simulink model "AerosondA_UAV_6DOF"  (R2021a)
settings: Solver=VariableStepAuto  StartTime=0.0  StopTime=20.0  RelTol=1e-3
InitFcn:
  | %%%%%%%%%%%%%%%%%%%%%%% Airframe Parameters %%%%%%%%%%%%%%%%%%%%%%%%%%%%%%%
  | 
  | m=13.5; % mass(kg)
  | Ix=0.8244; % Inertia along x axis (kg*m^2)
  | Iy=1.135; % Inertia along y axis (kg*m^2)
  | Iz=1.759; % Inertia along z axis (kg*m^2)
  | Ixy=0; % Inertia on xy plane (kg*m^2)
  | Iyz=0; % Inertia on yz plane (kg*m^2)
  | Ixz=0.1204; % Inertia on xz plane (kg*m^2)
  | I=[Ix -Ixy -Ixz;-Ixy Iy -Iyz;-Ixz -Iyz Iz]; % Inertia Matrix
  | S=0.55; % Surface Area (m^2)
  | b=2.8956; % Wingspan (m)
  | c=0.18994; % Chord (m)
  | Sprop=0.2027; % Propeller Surface Area (m^2)
  | k_motor=80; % Motor Constant
  | kTp=0; % Experimental Constant
  | k_omega=0; % Propeller Rotation Constant
  | rho_SL=1.225; % Sea Level air Density(kg/m^3)
  | TrimCondition(1)=-3.0373; % Elevator Trim At 100 m (degree)
  | TrimCondition(2)=0; % Aileron Trim At 100 m (degree)
  | TrimCondition(3)=0; % Rudder Trim At 100 m (degree)
  | TrimCondition(4)=0.45225; % Throttle Trim At 100 m
  | 
  | 
  | 
  | %%%%%%%%%%%%%%%%%%%%% Longitudinal Coefficients %%%%%%%%%%%%%%%%%%%%%%%%%%%
  | 
  | CL0=0.28;
  | CD0=0.03;
  | Cm0=-0.02338;
  | dCLdalpha=3.45;
  | dCDdalpha=0.3;
  | dCmdalpha=-0.38;
  | dCLdq=0;
  | dCDdq=0;
  | dCmdq=-3.6;
  | dCLdsigmaE=-0.36;
  | dCDdsigmaE=0;
  | dCmdsigmaE=-0.5;
  | Cprop=1;
  | M=50;
  | alpha_0=0.4712;
  | epsilon=0.1592;
  | dCDdp=0.0437;
  | dCndsigmaR=-0.032;
  | 
  | 
  | %%%%%%%%%%%%%%%%%%%%%%%% Lateral Coefficients %%%%%%%%%%%%%%%%%%%%%%%%%%%%%
  | 
  | Cy0=0;
  | Cl0=0;
  | Cn0=0;
  | dCydbeta=-0.98;
  | dCldbeta=-0.12;
  | dCndbeta=0.25;
  | dCydp=0;
  | dCldp=-0.26;
  | dCndp=0.022;
  | dCydr=0;
  | dCldr=0.14;
  | dCndr=-0.35;
  | dCydsigmaA=0;
  | dCldsigmaA=0.08;
  | dCndsigmaA=0.06;
  | dCydsigmaR=-0.17;
  | dCldsigmaR=-0.105;
undefined symbols (not defined in the file): TrimCondition
libraries: simulink_extras x3, aerolibutil x1
settings Model: Creator=hasre  LastModifiedBy=hasre

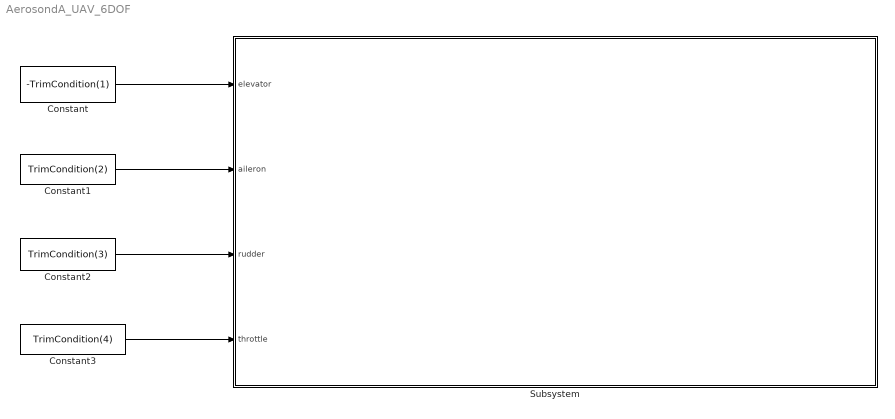
== system AerosondA_UAV_6DOF ==
  Constant : Constant  Value=-TrimCondition(1)
  Constant1 : Constant  Value=TrimCondition(2)
  Constant2 : Constant  Value=TrimCondition(3)
  Constant3 : Constant  Value=TrimCondition(4)
  Subsystem : Subsystem
  wires:
  Constant/1 -> Subsystem/1("elevator ")
  Constant1/1 -> Subsystem/2("aileron ")
  Constant2/1 -> Subsystem/3("rudder ")
  Constant3/1 -> Subsystem/4("throttle ")

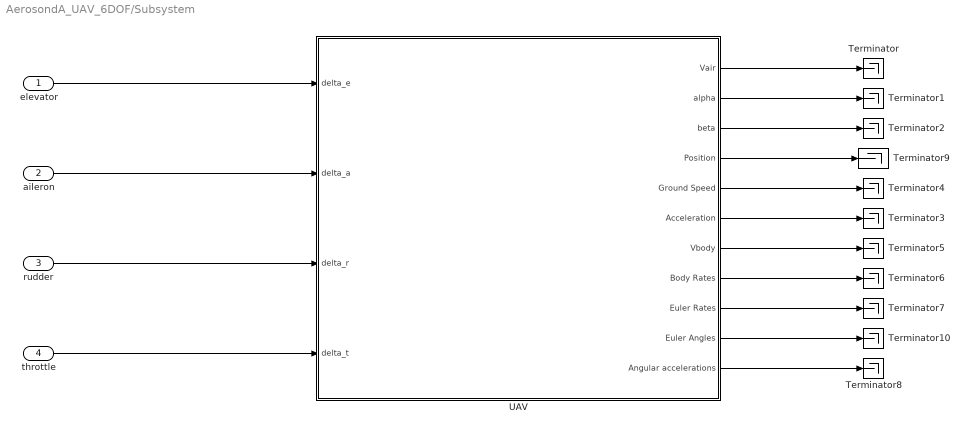
== system AerosondA_UAV_6DOF/Subsystem ==
  "elevator " : Inport
  "aileron " : Inport  Port=2
  "rudder " : Inport  Port=3
  "throttle " : Inport  Port=4
  Terminator{,1..10} (11 alike) : Terminator
  UAV : Subsystem
  wires:
  UAV/8(Body Rates) -> Terminator6/1
  UAV/6(Acceleration) -> Terminator3/1
  UAV/7(Vbody) -> Terminator5/1
  "elevator "/1 -> UAV/1(delta_e)
  UAV/3(beta) -> Terminator2/1
  "aileron "/1 -> UAV/2("delta_a ")
  UAV/4(Position) -> Terminator9/1
  UAV/1(Vair) -> Terminator/1
  UAV/11(Angular accelerations) -> Terminator8/1
  "throttle "/1 -> UAV/4(delta_t)
  UAV/2(alpha) -> Terminator1/1
  UAV/9(Euler Rates) -> Terminator7/1
  "rudder "/1 -> UAV/3(delta_r)
  UAV/5(Ground Speed) -> Terminator4/1
  UAV/10(Euler Angles) -> Terminator10/1

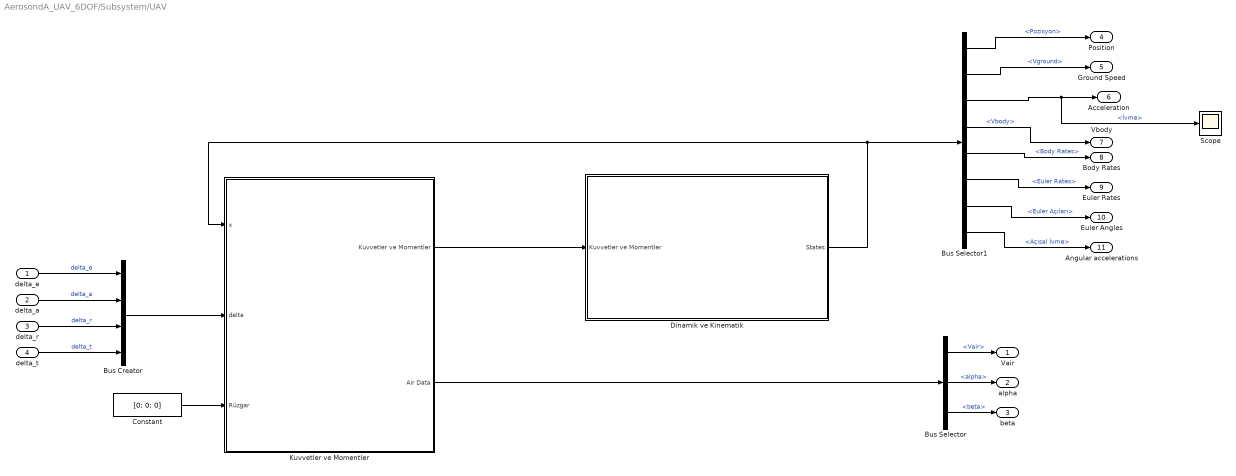
== system AerosondA_UAV_6DOF/Subsystem/UAV ==
  delta_e : Inport
  "delta_a " : Inport  Port=2
  delta_r : Inport  Port=3
  delta_t : Inport  Port=4
  Bus Creator : BusCreator  Inputs=4
  Bus Selector : BusSelector  OutputSignals=Vair,alpha,beta
  Bus Selector1 : BusSelector  OutputSignals=Pozisyon,Vground,İvme,Vbody,Body Rates,Euler Rates,Euler Açıları,Açısal İvme
  Constant : Constant  Value=[0; 0; 0]  VectorParams1D=off
  Dinamik ve Kinematik : Subsystem
  Kuvvetler ve Momentler : Subsystem
  Scope : Scope
  Vair : Outport
  alpha : Outport  Port=2
  beta : Outport  Port=3
  Position : Outport  Port=4
  Ground Speed : Outport  Port=5
  Acceleration : Outport  Port=6
  Vbody : Outport  Port=7
  Body Rates : Outport  Port=8
  Euler Rates : Outport  Port=9
  Euler Angles : Outport  Port=10
  Angular accelerations : Outport  Port=11
  wires:
  Kuvvetler ve Momentler/1(Kuvvetler ve Momentler) -> Dinamik ve Kinematik/1(Kuvvetler ve Momentler)
  delta_r/1 -> Bus Creator/3  "delta_r"
  delta_e/1 -> Bus Creator/1  "delta_e"
  Dinamik ve Kinematik/1(States) -> Kuvvetler ve Momentler/1("x "), Bus Selector1/1
  "delta_a "/1 -> Bus Creator/2  "delta_a"
  delta_t/1 -> Bus Creator/4  "delta_t"
  Bus Selector/2 -> alpha/1  "<alpha>"
  Bus Selector/1 -> Vair/1  "<Vair>"
  Kuvvetler ve Momentler/2(Air Data) -> Bus Selector/1
  Bus Selector/3 -> beta/1  "<beta>"
  Bus Creator/1 -> Kuvvetler ve Momentler/2("delta ")
  Constant/1 -> Kuvvetler ve Momentler/3(Rüzgar)
  Bus Selector1/1 -> Position/1  "<Pozisyon>"
  Bus Selector1/2 -> Ground Speed/1  "<Vground>"
  Bus Selector1/3 -> Scope/1, Acceleration/1  "<İvme>"
  Bus Selector1/4 -> Vbody/1  "<Vbody>"
  Bus Selector1/5 -> Body Rates/1  "<Body Rates>"
  Bus Selector1/6 -> Euler Rates/1  "<Euler Rates>"
  Bus Selector1/7 -> Euler Angles/1  "<Euler Açıları>"
  Bus Selector1/8 -> Angular accelerations/1  "<Açısal İvme>"

== system AerosondA_UAV_6DOF/Subsystem/UAV/Dinamik ve Kinematik ==
  Kuvvetler ve Momentler : Inport
  6 DOF Model : Subsystem
  Bus Creator : BusCreator  Inputs=9
  Bus Selector : BusSelector  OutputSignals=Kuvvetler,Momentler
  States : Outport
  wires:
  6 DOF Model/7(İvme (m/s2)) -> Bus Creator/7  "İvme"
  6 DOF Model/4(ωb (rad/s)) -> Bus Creator/4  "Body Rates"
  6 DOF Model/8(Earth Fixed Pos. (m)) -> Bus Creator/8  "Pozisyon"
  6 DOF Model/9(DCMvb) -> Bus Creator/9  "Euler Matrix"
  6 DOF Model/1("ϕ θ ψ (rad)  ") -> Bus Creator/1  "Euler Açıları"
  6 DOF Model/3("Vb (m/s) ") -> Bus Creator/3  "Vbody"
  6 DOF Model/5(dωb/dt) -> Bus Creator/5  "Açısal İvme"
  6 DOF Model/6(Vg) -> Bus Creator/6  "Vground"
  Kuvvetler ve Momentler/1 -> Bus Selector/1
  Bus Selector/2 -> 6 DOF Model/2(Moment)  "<Momentler>"
  Bus Selector/1 -> 6 DOF Model/1(Kuvvet)  "<Kuvvetler>"
  6 DOF Model/2(ϕ θ ψ rates (rad/s)) -> Bus Creator/2  "Euler Rates"
  Bus Creator/1 -> States/1

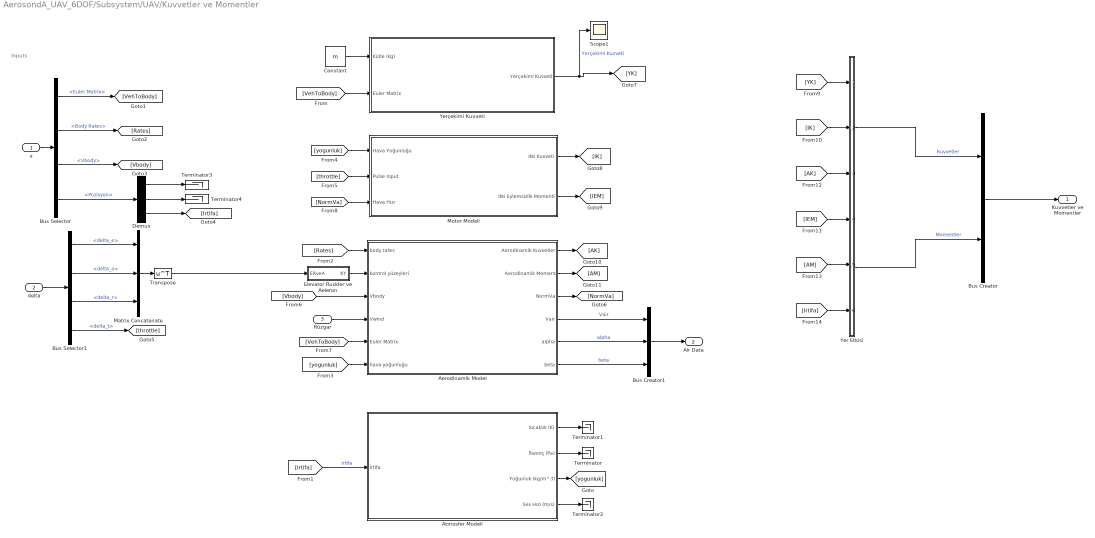
== system AerosondA_UAV_6DOF/Subsystem/UAV/Kuvvetler ve Momentler ==
  note: Inputs
  "x " : Inport
  "delta " : Inport  Port=2
  Rüzgar : Inport  Port=3
  Aerodinamik Model : Subsystem
  Atmosfer Modeli : Subsystem
  Bus Creator : BusCreator  Inputs=2
  Bus Creator1 : BusCreator  Inputs=3
  Bus Selector : BusSelector  OutputSignals=Euler Matrix,Body Rates,Vbody,Pozisyon
  Bus Selector1 : BusSelector  OutputSignals=delta_e,delta_a,delta_r,delta_t
  Constant : Constant  Value=m
  Demux : Demux  Outputs=3
  Elevator Rudder ve Aeleron : Subsystem
  Matrix Concatenate : Concatenate  NumInputs=3  Mode=Multidimensional array  ConcatenateDimension=2
  Motor Modeli : Subsystem
  Scope1 : Scope
  Terminator{,1..4} (5 alike) : Terminator
  Transpose : Math  Operator=transpose  SaturateOnIntegerOverflow=on
  "Yer Etkisi " : Subsystem
  Yerçekimi Kuvveti : Subsystem
  Kuvvetler ve Momentler : Outport
  Air Data : Outport  Port=2
  wires:
  Atmosfer Modeli/3(Yoğunluk (kg/m^3)) -> [yogunluk]
  [Irtifa] -> Atmosfer Modeli/1("İrtifa ")  "irtifa"
  [throttle] -> Motor Modeli/2("Pulse Input ")
  Atmosfer Modeli/4(Ses Hızı (m/s)) -> Terminator2/1
  Constant/1 -> Yerçekimi Kuvveti/1(Kütle (kg))
  [VehToBody] -> Yerçekimi Kuvveti/2(Euler Matrix)
  Elevator Rudder ve Aeleron/1(KY) -> Aerodinamik Model/2(kontrol yüzeyleri)
  [Rates] -> Aerodinamik Model/1("body rates ")
  Atmosfer Modeli/2(Basınç (Pa)) -> Terminator/1
  [yogunluk] -> Motor Modeli/1(Hava Yoğunluğu)
  Atmosfer Modeli/1(Sıcaklık (K)) -> Terminator1/1
  [yogunluk] -> Aerodinamik Model/6("hava yoğunluğu ")
  "Yer Etkisi "/2(Out2) -> Bus Creator/2  "Momentler"
  "Yer Etkisi "/1(Out1) -> Bus Creator/1  "Kuvvetler"
  Bus Creator/1 -> Kuvvetler ve Momentler/1
  "x "/1 -> Bus Selector/1
  Bus Selector/1 -> [VehToBody]  "<Euler Matrix>"
  Bus Selector/2 -> [Rates]  "<Body Rates>"
  Bus Selector/3 -> [Vbody]  "<Vbody>"
  Rüzgar/1 -> Aerodinamik Model/4("Vwind ")
  "delta "/1 -> Bus Selector1/1
  Bus Selector1/1 -> Matrix Concatenate/1  "<delta_e>"
  Bus Selector1/2 -> Matrix Concatenate/2  "<delta_a>"
  Bus Selector1/3 -> Matrix Concatenate/3  "<delta_r>"
  Matrix Concatenate/1 -> Transpose/1
  Bus Selector1/4 -> [throttle]  "<delta_t>"
  Transpose/1 -> Elevator Rudder ve Aeleron/1(ERveA)
  [Vbody] -> Aerodinamik Model/3("Vbody ")
  Bus Selector/4 -> Demux/1  "<Pozisyon>"
  [VehToBody] -> Aerodinamik Model/5("Euler Matrix ")
  Aerodinamik Model/5(alpha) -> Bus Creator1/2  "alpha"
  Aerodinamik Model/4(Vair) -> Bus Creator1/1  "Vair"
  Aerodinamik Model/6(beta) -> Bus Creator1/3  "beta"
  Bus Creator1/1 -> Air Data/1
  [NormVa] -> Motor Modeli/3(Hava Hızı)
  Aerodinamik Model/3(NormVa) -> [NormVa]
  Yerçekimi Kuvveti/1("Yerçekimi Kuvveti ") -> Scope1/1, [YK]  "Yerçekimi Kuvveti"
  Motor Modeli/1("İtki Kuvveti ") -> [IK]
  Motor Modeli/2(İtki Eylemsizlik Momenti) -> [IEM]
  Aerodinamik Model/1(Aerodinamik Kuvvetler) -> [AK]
  Aerodinamik Model/2(Aerodinamik Moment) -> [AM]
  [YK] -> "Yer Etkisi "/1(In1)
  [IK] -> "Yer Etkisi "/2(In2)
  [IEM] -> "Yer Etkisi "/4(In4)
  [AK] -> "Yer Etkisi "/3(In3)
  [AM] -> "Yer Etkisi "/5(In5)
  Demux/1 -> Terminator3/1
  Demux/2 -> Terminator4/1
  Demux/3 -> [Irtifa]
  [Irtifa] -> "Yer Etkisi "/6("İrtifa ")

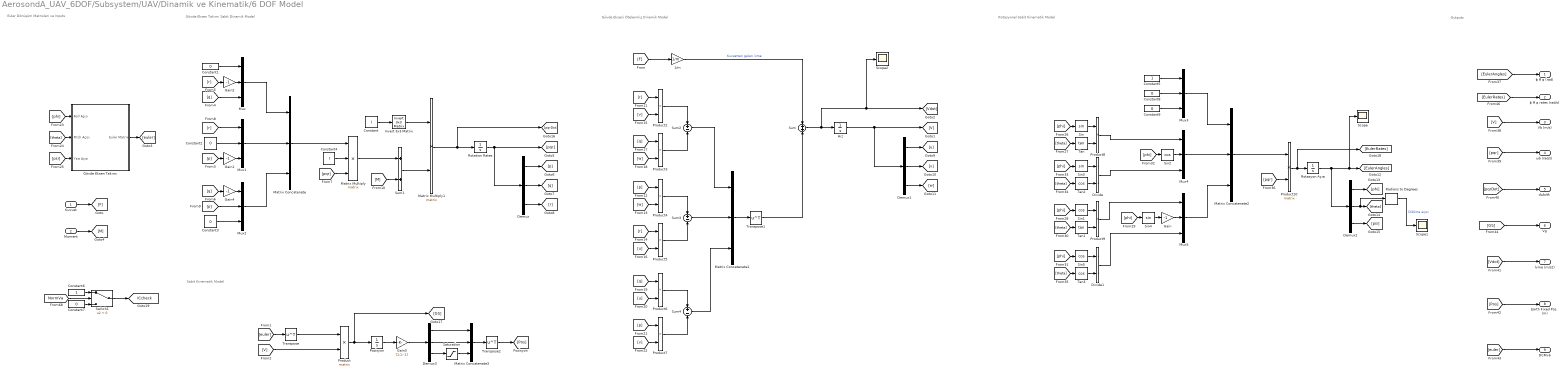
== system AerosondA_UAV_6DOF/Subsystem/UAV/Dinamik ve Kinematik/6 DOF Model ==
  note: Euler Dönüşüm Matrisleri ve
      |  Inputs
  note: Gövde Eksen Takımı Sabit Dinamik Model
  note: Sabit Kinematik Model
  note: Gövde Ekseni Ötelenmiş Dinamik Model
  note: Rotasyonel Sabit Kinematik Model
  note: Outputs
  Kuvvet : Inport
  Moment : Inport  Port=2
  "1/m " : Gain  Gain=1/m
  Constant : Constant  Value=I  VectorParams1D=off
  Constant{1..3,8..9} (5 alike) : Constant  Value=0  VectorParams1D=off
  Constant4 : Constant  Value=I  VectorParams1D=off
  Constant5 : Constant  VectorParams1D=off
  Constant6 : Constant
  Constant7 : Constant  Value=0
  Demux{,1..3} (4 alike) : Demux  Outputs=3
  Divide : Product  Inputs=*/
  Divide1 : Product  Inputs=*/
  Gain{,1..2,4} (4 alike) : Gain  Gain=-1
  Gain3 : Gain  Gain=[1;1;-1]
  "Gövde Eksen Takımı " : Subsystem
  Hız : Integrator  InitialCondition=[34.8015;0;0]  ZeroCross=off
  Invert 3x3 Matrix : aerolibutil/Invert  3x3 Matrix
  Matrix Concatenate{,1..3} (4 alike) : Concatenate  NumInputs=3  Mode=Multidimensional array  ConcatenateDimension=2
  Matrix Multiply : Product  Inputs=3  Multiplication=Matrix(*)
  Matrix Multiply1 : Product  Multiplication=Matrix(*)
  Mux{,1..5} (6 alike) : Mux  Inputs=3
  Pozisyon : Integrator  InitialCondition=[0;0;-100]
  Product : Product  Multiplication=Matrix(*)
  Product10 : Product  Multiplication=Matrix(*)
  Product{2..9} (8 alike) : Product
  Radians to Degrees : simulink_extras/Transformations/Radians to Degrees
  Rotasyon Açısı : Integrator
  Rotation Rates : Integrator
  Saturation : Saturate  UpperLimit=inf  LowerLimit=0
  Scope : Scope
  Scope1 : Scope
  Scope2 : Scope
  Sin : Trigonometry
  Sin1 : Trigonometry  Operator=cos
  Sin2 : Trigonometry  Operator=cos
  Sin3 : Trigonometry
  Sin4 : Trigonometry
  Sin5 : Trigonometry  Operator=cos
  Sum : Sum
  Sum1 : Sum
  Sum2 : Sum  Inputs=+-
  Sum3 : Sum  Inputs=+-
  Sum4 : Sum  Inputs=+-
  Switch1 : Switch  Criteria=u2 > Threshold
  Tan : Trigonometry  Operator=tan
  Tan1 : Trigonometry  Operator=tan
  Tan2 : Trigonometry  Operator=cos
  Tan3 : Trigonometry  Operator=cos
  Transpose : Math  Operator=transpose  SaturateOnIntegerOverflow=on
  Transpose1 : Math  Operator=transpose  SaturateOnIntegerOverflow=on
  Transpose2 : Math  Operator=transpose  SaturateOnIntegerOverflow=on
  "ϕ θ ψ (rad)  " : Outport
  ϕ θ ψ rates (rad/s) : Outport  Port=2
  "Vb (m/s) " : Outport  Port=3
  ωb (rad/s) : Outport  Port=4
  dωb/dt : Outport  Port=5
  Vg : Outport  Port=6
  İvme (m/s2) : Outport  Port=7
  Earth Fixed Pos. (m) : Outport  Port=8
  DCMvb : Outport  Port=9
  tag scope: ICcheck=global
  wires:
  Kuvvet/1 -> [F]
  [F] -> "1/m "/1
  Sum/1 -> Scope2/1, [Vdot], Hız/1
  "Gövde Eksen Takımı "/1("Euler Matrix ") -> [euler]
  Moment/1 -> [M]
  [p] -> Gain1/1
  Constant1/1 -> Mux/1
  [pqr] -> Matrix Multiply/3
  Demux/3 -> [r]
  Demux/2 -> [q]
  Invert 3x3 Matrix/1 -> Matrix Multiply1/1
  Constant2/1 -> Mux1/2
  [p] -> Mux2/2
  Matrix Multiply/1 -> Sum1/1
  Mux2/1 -> Matrix Concatenate/3
  [q] -> Gain4/1
  Sum1/1 -> Matrix Multiply1/2
  Matrix Multiply1/1 -> [pqrDot], Rotation Rates/1
  Demux/1 -> [p]
  Mux1/1 -> Matrix Concatenate/2
  Gain2/1 -> Mux/2
  [M] -> Sum1/2
  Constant3/1 -> Mux2/3
  [r] -> Gain2/1
  Rotation Rates/1 -> Demux/1, [pqr]
  Constant4/1 -> Matrix Multiply/2
  [q] -> Mux/3
  Mux/1 -> Matrix Concatenate/1
  Matrix Concatenate/1 -> Matrix Multiply/1
  Gain1/1 -> Mux1/3
  [r] -> Mux1/1
  Gain4/1 -> Mux2/1
  Constant/1 -> Invert 3x3 Matrix/1
  Hız/1 -> Demux1/1, [V]
  Demux1/1 -> [u]
  Demux1/2 -> [v]
  Demux1/3 -> [w]
  [v] -> Product2/2
  [r] -> Product2/1
  [q] -> Product3/1
  [w] -> Product3/2
  Product2/1 -> Sum2/1
  Product3/1 -> Sum2/2
  Product5/1 -> Sum3/2
  Product4/1 -> Sum3/1
  [u] -> Product5/2
  [r] -> Product5/1
  [p] -> Product4/1
  [w] -> Product4/2
  [u] -> Product6/2
  [q] -> Product6/1
  [p] -> Product7/1
  [v] -> Product7/2
  Product6/1 -> Sum4/1
  Product7/1 -> Sum4/2
  Sum2/1 -> Matrix Concatenate1/1
  Sum3/1 -> Matrix Concatenate1/2
  Sum4/1 -> Matrix Concatenate1/3
  Matrix Concatenate1/1 -> Transpose1/1
  Transpose1/1 -> Sum/2
  "1/m "/1 -> Sum/1  "Kuvvetten gelen ivme"
  Pozisyon/1 -> Gain3/1
  [euler] -> Transpose/1
  Product/1 -> [GS], Pozisyon/1
  [V] -> Product/2
  Transpose/1 -> Product/1
  Rotasyon Açısı/1 -> Demux2/1, Scope/1, [EulerAngles]
  Demux2/1 -> [phi]
  Demux2/2 -> Radians to Degrees/1, [theta]
  Demux2/3 -> [psi]
  [phi] -> "Gövde Eksen Takımı "/1("Roll Açısı ")
  [theta] -> "Gövde Eksen Takımı "/2("Pitch Açısı ")
  [psi] -> "Gövde Eksen Takımı "/3("Yaw Açısı ")
  Constant5/1 -> Mux3/1
  Mux5/1 -> Matrix Concatenate2/3
  Mux3/1 -> Matrix Concatenate2/1
  Mux4/1 -> Matrix Concatenate2/2
  Matrix Concatenate2/1 -> Product10/1
  Product9/1 -> Mux5/1
  Constant9/1 -> Mux3/3
  Constant8/1 -> Mux3/2
  [theta] -> Tan/1
  Tan/1 -> Product8/2
  Sin/1 -> Product8/1
  [phi] -> Sin/1
  [phi] -> Sin1/1
  Sin1/1 -> Product9/1
  Tan1/1 -> Product9/2
  [theta] -> Tan1/1
  Product8/1 -> Mux4/1
  Sin2/1 -> Mux4/2
  [phi] -> Sin2/1
  [theta] -> Tan2/1
  Tan2/1 -> Divide/2
  Sin3/1 -> Divide/1
  [phi] -> Sin3/1
  Divide/1 -> Mux4/3
  [phi] -> Sin4/1
  Sin4/1 -> Gain/1
  Gain/1 -> Mux5/2
  Divide1/1 -> Mux5/3
  [phi] -> Sin5/1
  Sin5/1 -> Divide1/1
  Tan3/1 -> Divide1/2
  [theta] -> Tan3/1
  [pqr] -> Product10/2
  Product10/1 -> [EulerRates], Rotasyon Açısı/1
  [EulerAngles] -> "ϕ θ ψ (rad)  "/1
  [V] -> "Vb (m/s) "/1
  [pqr] -> ωb (rad/s)/1
  [pqrDot] -> dωb/dt/1
  [Vdot] -> İvme (m/s2)/1
  [Pos] -> Earth Fixed Pos. (m)/1
  [euler] -> DCMvb/1
  [GS] -> Vg/1
  [EulerRates] -> ϕ θ ψ rates (rad/s)/1
  Gain3/1 -> Demux3/1
  Demux3/1 -> Matrix Concatenate3/1
  Demux3/2 -> Matrix Concatenate3/2
  Demux3/3 -> Saturation/1
  Saturation/1 -> Matrix Concatenate3/3
  Matrix Concatenate3/1 -> Transpose2/1
  Transpose2/1 -> [Pos]
  Switch1/1 -> [ICcheck]
  Constant6/1 -> Switch1/1
  [NormVa] -> Switch1/2
  Constant7/1 -> Switch1/3
  Radians to Degrees/1 -> Scope1/1  "Dikilme açısı"

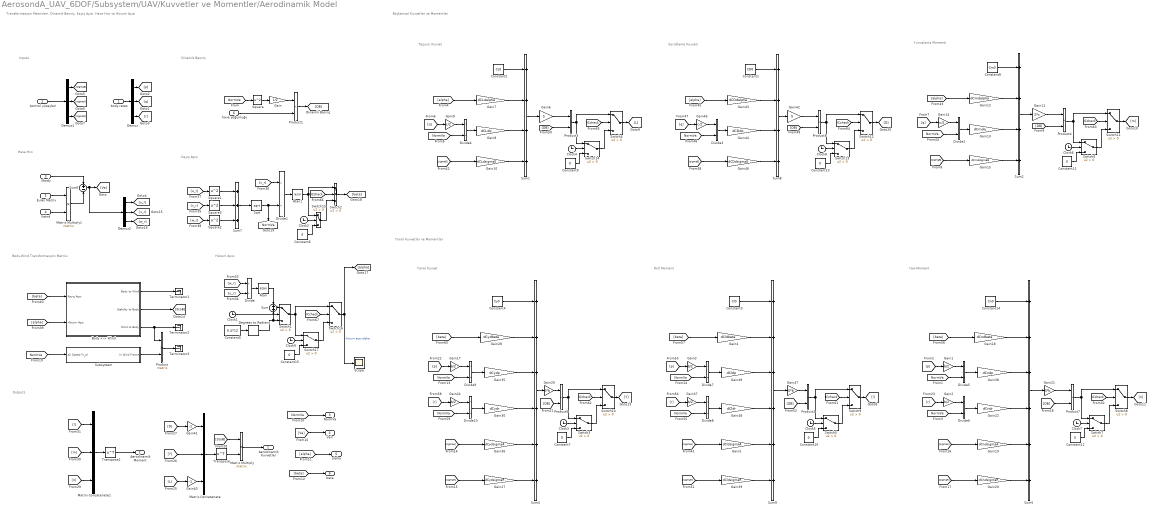
== system AerosondA_UAV_6DOF/Subsystem/UAV/Kuvvetler ve Momentler/Aerodinamik Model ==
  note: Transformasyon Matrisleri, Dinamik Basınç, Kayış Açısı, Hava Hızı ve Hücum Açısı
  note: Boylamsal Kuvvetler ve Momentler
  note: Yunuslama Momenti
  note: Yanal Kuvvetler ve Momentler
  note: Yaw Moment
  note: Hava Hızı
  note: Hücum Açısı
  note: Kayış Açısı
  note: Body-Wind Transformasyon Matrisi
  note: Dinamik Basınç
  note: Inputs
  note: Outputs
  note: Sürükleme Kuvveti
  note: Taşıyıcı Kuvvet
  note: Roll Moment
  note: Yanal Kuvvet
  "body rates " : Inport
  kontrol yüzeyleri : Inport  Port=2
  "Vbody " : Inport  Port=3
  "Vwind " : Inport  Port=4
  "Euler Matrix " : Inport  Port=5
  "hava yoğunluğu " : Inport  Port=6
  Atan : Trigonometry  Operator=atan
  Atan1 : Trigonometry  Operator=asin
  "Body <-> Wind " : Subsystem
  Clock{1..9} (9 alike) : Clock
      settings: Decimation=20
  Constant1 : Constant  Value=CD0
  Constant{6..7,9..13,15} (8 alike) : Constant  Value=0
  Constant14 : Constant  Value=Cn0  VectorParams1D=off
  Constant2 : Constant  Value=CL0  VectorParams1D=off
  Constant3 : Constant  Value=Cl0  VectorParams1D=off
  Constant4 : Constant  Value=Cy0  VectorParams1D=off
  Constant5 : Constant  Value=0.4712
  Constant8 : Constant  Value=Cm0  VectorParams1D=off
  Degrees to Radians : simulink_extras/Transformations/Degrees to Radians
  Demux : Demux  Outputs=3
  Demux1 : Demux  Outputs=3
  Demux2 : Demux  Outputs=3
  Divide{,1..10} (11 alike) : Product  Inputs=*/
  Gain : Gain  Gain=1/2
  Gain{1..3,17,24,37} (6 alike) : Gain  Gain=b/2
  Gain10 : Gain  Gain=dCLdsigmaE
  Gain11 : Gain  Gain=S*c
  Gain12 : Gain  Gain=dCmdalpha
  Gain13 : Gain  Gain=dCmdq
  Gain14 : Gain  Gain=c/2
  Gain15 : Gain  Gain=dCmdsigmaE
  Gain18 : Gain  Gain=dCndbeta
  Gain19 : Gain  Gain=dCndsigmaA
  Gain20 : Gain  Gain=dCndsigmaR
  Gain21 : Gain  Gain=S*b
  Gain22 : Gain  Gain=dCndr
  Gain27 : Gain  Gain=dCydsigmaR
  Gain28 : Gain  Gain=dCydbeta
  Gain29 : Gain  Gain=S*b
  Gain30 : Gain  Gain=dCydr
  Gain35 : Gain  Gain=dCydp
  Gain36 : Gain  Gain=dCydsigmaA
  Gain38 : Gain  Gain=dCndp
  Gain39 : Gain  Gain=dCldsigmaR
  Gain4 : Gain  Gain=dCldbeta
  Gain40 : Gain  Gain=-1
  Gain41 : Gain  Gain=-1
  Gain42 : Gain  Gain=S
  Gain43 : Gain  Gain=dCDdalpha
  Gain44 : Gain  Gain=dCDdq
  Gain45 : Gain  Gain=c/2
  Gain46 : Gain  Gain=dCDdsigmaE
  Gain47 : Gain  Gain=S*b
  Gain48 : Gain  Gain=dCldr
  Gain49 : Gain  Gain=dCldp
  Gain5 : Gain  Gain=dCldsigmaA
  Gain6 : Gain  Gain=S
  Gain7 : Gain  Gain=dCLdalpha
  Gain8 : Gain  Gain=dCLdq
  Gain9 : Gain  Gain=c/2
  Matrix Concatenate : Concatenate  NumInputs=3  Mode=Multidimensional array  ConcatenateDimension=2
  Matrix Concatenate1 : Concatenate  NumInputs=3  Mode=Multidimensional array  ConcatenateDimension=2
  Matrix Multiply : Product  Multiplication=Matrix(*)
  Matrix Multiply1 : Product  Multiplication=Matrix(*)
  Product : Product  Multiplication=Matrix(*)
  Product{1..4,6..8} (7 alike) : Product
  Scope : Scope
  Sqrt : Sqrt  SaturateOnIntegerOverflow=on
  Square{,1..3} (4 alike) : Math  Operator=square  SaturateOnIntegerOverflow=on
  Subsystem : Subsystem
  Sum : Sum
  Sum1 : Sum  Inputs=++++
  Sum2 : Sum  Inputs=++++
  Sum4 : Sum  Inputs=++++++
  Sum5 : Sum  Inputs=++++++
  Sum6 : Sum  Inputs=+-
  Sum7 : Sum  Inputs=+++
  Sum8 : Sum  Inputs=++++
  Sum9 : Sum  Inputs=++++++
  Switch{1..17} (17 alike) : Switch  Criteria=u2 > Threshold
  Terminator1 : Terminator
  Terminator2 : Terminator
  Terminator3 : Terminator
  Transpose : Math  Operator=transpose  SaturateOnIntegerOverflow=on
  Transpose1 : Math  Operator=transpose  SaturateOnIntegerOverflow=on
  Aerodinamik Kuvvetler : Outport
  Aerodinamik Moment : Outport  Port=2
  NormVa : Outport  Port=3
  Vair : Outport  Port=4
  alpha : Outport  Port=5
  beta : Outport  Port=6
  tag scope: NormVa=global
  wires:
  "body rates "/1 -> Demux/1
  Demux/2 -> [q]
  Demux/1 -> [p]
  Demux/3 -> [r]
  kontrol yüzeyleri/1 -> Demux1/1
  Demux1/1 -> [sigmaE]
  Demux1/2 -> [sigmaA]
  Demux1/3 -> [sigmaR]
  [alpha] -> Gain12/1
  [q] -> Gain14/1
  [sigmaE] -> Gain15/1
  Gain15/1 -> Sum2/4
  Gain13/1 -> Sum2/3
  Gain12/1 -> Sum2/2
  Constant8/1 -> Sum2/1
  Sum2/1 -> Gain11/1
  Gain11/1 -> Product4/1
  [DB] -> Product4/2
  Product7/1 -> Switch8/1, Switch7/1
  [DB] -> Product7/2
  Gain21/1 -> Product7/1
  Sum5/1 -> Gain21/1
  Constant14/1 -> Sum5/1
  Gain18/1 -> Sum5/2
  Gain19/1 -> Sum5/5
  Gain20/1 -> Sum5/6
  [sigmaR] -> Gain20/1
  [beta] -> Gain18/1
  Gain38/1 -> Sum5/3
  Gain22/1 -> Sum5/4
  Divide5/1 -> Gain38/1
  Divide6/1 -> Gain22/1
  [sigmaA] -> Gain19/1
  [L] -> Gain40/1
  Gain40/1 -> Matrix Concatenate/3
  [Y] -> Matrix Concatenate/2
  [D] -> Gain41/1
  Gain41/1 -> Matrix Concatenate/1
  Matrix Concatenate/1 -> Transpose/1
  Transpose/1 -> Matrix Multiply/2
  [StoB] -> Matrix Multiply/1
  Matrix Multiply/1 -> Aerodinamik Kuvvetler/1
  Transpose1/1 -> Aerodinamik Moment/1
  Matrix Concatenate1/1 -> Transpose1/1
  [l] -> Matrix Concatenate1/1
  [m] -> Matrix Concatenate1/2
  [n] -> Matrix Concatenate1/3
  "Vbody "/1 -> Sum6/1
  Sum6/1 -> Demux2/1, [Va]
  "Euler Matrix "/1 -> Matrix Multiply1/1
  "Vwind "/1 -> Matrix Multiply1/2
  Matrix Multiply1/1 -> Sum6/2
  Demux2/1 -> [u_r]
  Demux2/2 -> [v_r]
  Demux2/3 -> [w_r]
  [w_r] -> Divide/1
  [u_r] -> Divide/2
  Divide/1 -> Atan/1
  Divide1/1 -> Atan1/1
  [w_r] -> Square2/1
  [u_r] -> Square1/1
  Square1/1 -> Sum7/1
  Square2/1 -> Sum7/3
  Square3/1 -> Sum7/2
  [v_r] -> Square3/1
  Sum7/1 -> Sqrt/1
  Sqrt/1 -> Divide1/2, [NormVa]
  [v_r] -> Divide1/1
  "Body <-> Wind "/1("Body to Wind ") -> Terminator1/1
  [beta] -> "Body <-> Wind "/1("Kayış Açısı ")
  [NormVa] -> Subsystem/1(Air Speed (V_a))
  "Body <-> Wind "/3(Wind to Body) -> Terminator2/1, Product/1
  Subsystem/1(In Wind Frame) -> Product/2
  [alpha] -> "Body <-> Wind "/2("Hücum Açısı ")
  Product/1 -> Terminator3/1
  "Body <-> Wind "/2(Stability to Body) -> [StoB]
  "hava yoğunluğu "/1 -> Product1/2
  Square/1 -> Gain/1
  [NormVa] -> Square/1
  Gain/1 -> Product1/1
  Product1/1 -> [DB]
  Divide2/1 -> Gain13/1
  Gain14/1 -> Divide2/1
  [NormVa] -> Divide2/2
  [NormVa] -> Divide3/2
  Gain45/1 -> Divide3/1
  Divide3/1 -> Gain44/1
  [DB] -> Product8/2
  Gain42/1 -> Product8/1
  Sum8/1 -> Gain42/1
  Constant1/1 -> Sum8/1
  Gain43/1 -> Sum8/2
  Gain44/1 -> Sum8/3
  Gain46/1 -> Sum8/4
  [sigmaE] -> Gain46/1
  [q] -> Gain45/1
  [alpha] -> Gain43/1
  [alpha] -> Gain7/1
  [q] -> Gain9/1
  [sigmaE] -> Gain10/1
  Gain10/1 -> Sum1/4
  Gain8/1 -> Sum1/3
  Gain7/1 -> Sum1/2
  Constant2/1 -> Sum1/1
  Sum1/1 -> Gain6/1
  Gain6/1 -> Product3/1
  [DB] -> Product3/2
  Divide4/1 -> Gain8/1
  Gain9/1 -> Divide4/1
  [NormVa] -> Divide4/2
  [NormVa] -> Divide5/2
  Gain1/1 -> Divide5/1
  [p] -> Gain1/1
  [r] -> Gain2/1
  Gain2/1 -> Divide6/1
  [NormVa] -> Divide6/2
  [NormVa] -> Divide8/2
  Gain37/1 -> Divide8/1
  [r] -> Gain37/1
  [p] -> Gain3/1
  Gain3/1 -> Divide7/1
  [NormVa] -> Divide7/2
  [sigmaA] -> Gain5/1
  Divide8/1 -> Gain48/1
  Divide7/1 -> Gain49/1
  Gain48/1 -> Sum9/4
  Gain49/1 -> Sum9/3
  [beta] -> Gain4/1
  [sigmaR] -> Gain39/1
  Gain39/1 -> Sum9/6
  Gain5/1 -> Sum9/5
  Gain4/1 -> Sum9/2
  Constant3/1 -> Sum9/1
  Sum9/1 -> Gain47/1
  [DB] -> Product6/2
  Gain29/1 -> Product6/1
  Sum4/1 -> Gain29/1
  Constant4/1 -> Sum4/1
  Gain28/1 -> Sum4/2
  Gain36/1 -> Sum4/5
  Gain27/1 -> Sum4/6
  [sigmaR] -> Gain27/1
  [beta] -> Gain28/1
  Gain35/1 -> Sum4/3
  Gain30/1 -> Sum4/4
  Divide9/1 -> Gain35/1
  Divide10/1 -> Gain30/1
  [sigmaA] -> Gain36/1
  [NormVa] -> Divide9/2
  Gain17/1 -> Divide9/1
  [p] -> Gain17/1
  [r] -> Gain24/1
  Gain24/1 -> Divide10/1
  [NormVa] -> Divide10/2
  [Va] -> Vair/1
  [alpha] -> alpha/1
  [beta] -> beta/1
  [NormVa] -> NormVa/1
  Constant5/1 -> Degrees to Radians/1
  Clock1/1 -> Switch1/2
  Switch2/1 -> [beta]
  Switch4/1 -> [L]
  Switch11/1 -> [m]
  Constant12/1 -> Switch7/3
  Clock7/1 -> Switch7/2
  Degrees to Radians/1 -> Sum/2, Switch1/3
  Sum/1 -> Switch1/1
  Atan/1 -> Sum/1
  [ICcheck] -> Switch8/2
  Switch7/1 -> Switch8/3
  Switch8/1 -> [n]
  Switch9/1 -> [l]
  [ICcheck] -> Switch9/2
  Switch5/1 -> Switch9/3
  Clock5/1 -> Switch5/2
  [DB] -> Product2/2
  Constant10/1 -> Switch5/3
  Gain47/1 -> Product2/1
  Product2/1 -> Switch9/1, Switch5/1
  Switch10/1 -> [Y]
  Constant7/1 -> Switch3/3
  Switch3/1 -> Switch10/3
  Clock3/1 -> Switch3/2
  [ICcheck] -> Switch10/2
  Product6/1 -> Switch10/1, Switch3/1
  Constant11/1 -> Switch6/3
  Switch6/1 -> Switch11/3
  Clock6/1 -> Switch6/2
  [ICcheck] -> Switch11/2
  Product4/1 -> Switch11/1, Switch6/1
  Product8/1 -> Switch12/1, Switch13/1
  Switch13/1 -> Switch12/3
  Constant13/1 -> Switch13/3
  Switch12/1 -> [D]
  Clock8/1 -> Switch13/2
  [ICcheck] -> Switch12/2
  Product3/1 -> Switch4/1, Switch14/1
  Switch14/1 -> Switch4/3
  Constant9/1 -> Switch14/3
  Clock4/1 -> Switch14/2
  [ICcheck] -> Switch4/2
  Atan1/1 -> Switch2/1, Switch15/1
  Switch15/1 -> Switch2/3
  Constant6/1 -> Switch15/3
  Clock2/1 -> Switch15/2
  [ICcheck] -> Switch2/2
  Switch1/1 -> Switch16/1, Switch17/1
  Switch17/1 -> Switch16/3
  Constant15/1 -> Switch17/3
  Switch16/1 -> Scope/1, [alpha]  "hücum açısı alpha"
  Clock9/1 -> Switch17/2
  [ICcheck] -> Switch16/2

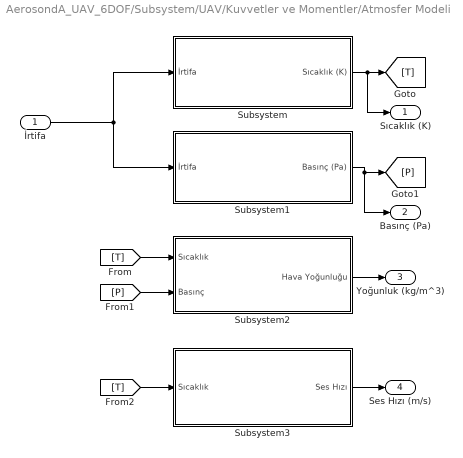
== system AerosondA_UAV_6DOF/Subsystem/UAV/Kuvvetler ve Momentler/Atmosfer Modeli ==
  "İrtifa " : Inport
  Subsystem : Subsystem
  Subsystem1 : Subsystem
  Subsystem2 : Subsystem
  Subsystem3 : Subsystem
  Sıcaklık (K) : Outport
  Basınç (Pa) : Outport  Port=2
  Yoğunluk (kg/m^3) : Outport  Port=3
  Ses Hızı (m/s) : Outport  Port=4
  wires:
  Subsystem/1(Sıcaklık (K)) -> Sıcaklık (K)/1, [T]
  Subsystem1/1(Basınç (Pa)) -> Basınç (Pa)/1, [P]
  [T] -> Subsystem2/1("Sıcaklık ")
  [P] -> Subsystem2/2(Basınç)
  [T] -> Subsystem3/1("Sıcaklık ")
  Subsystem2/1(Hava Yoğunluğu) -> Yoğunluk (kg/m^3)/1
  Subsystem3/1(Ses Hızı) -> Ses Hızı (m/s)/1
  "İrtifa "/1 -> Subsystem1/1("İrtifa "), Subsystem/1("İrtifa ")

== system AerosondA_UAV_6DOF/Subsystem/UAV/Kuvvetler ve Momentler/Elevator Rudder ve Aeleron ==
  ERveA : Inport
  Aileron Modeli : Subsystem
  Degrees to Radians : simulink_extras/Transformations/Degrees to Radians
  Demux : Demux  Outputs=3
  Elevator Modeli : Subsystem
  Matrix Concatenate : Concatenate  NumInputs=3  Mode=Multidimensional array  ConcatenateDimension=2
  Rudder Modeli : Subsystem
  Scope : Scope
  Transpose : Math  Operator=transpose  SaturateOnIntegerOverflow=on
  KY : Outport
  wires:
  Demux/3 -> Rudder Modeli/1(Rudder Açısı (İstenen))
  Demux/2 -> Aileron Modeli/1("Aileron Açısı (İstenen) ")
  Demux/1 -> Elevator Modeli/1(Elevator Açısı (İstenen))
  ERveA/1 -> Demux/1
  Rudder Modeli/1(Rudder Açısı) -> Matrix Concatenate/3
  Aileron Modeli/1("Aileron Açısı ") -> Matrix Concatenate/2
  Elevator Modeli/1(Elevator Açısı) -> Matrix Concatenate/1
  Matrix Concatenate/1 -> Transpose/1
  Transpose/1 -> Degrees to Radians/1
  Degrees to Radians/1 -> Scope/1, KY/1

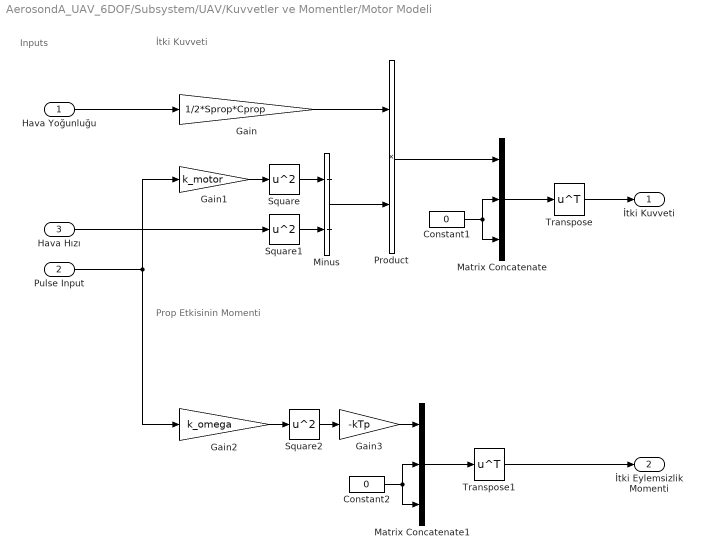
== system AerosondA_UAV_6DOF/Subsystem/UAV/Kuvvetler ve Momentler/Motor Modeli ==
  note: Inputs
  note: İtki Kuvveti
  note: Prop Etkisinin Momenti
  Hava Yoğunluğu : Inport
  "Pulse Input " : Inport  Port=2
  Hava Hızı : Inport  Port=3
  Constant1 : Constant  Value=0
  Constant2 : Constant  Value=0
  Gain : Gain  Gain=1/2*Sprop*Cprop
  Gain1 : Gain  Gain=k_motor
  Gain2 : Gain  Gain=k_omega
  Gain3 : Gain  Gain=-kTp
  Matrix Concatenate : Concatenate  NumInputs=3  Mode=Multidimensional array  ConcatenateDimension=2
  Matrix Concatenate1 : Concatenate  NumInputs=3  Mode=Multidimensional array  ConcatenateDimension=2
  Minus : Sum  Inputs=+-
  Product : Product
  Square : Math  Operator=square  SaturateOnIntegerOverflow=on
  Square1 : Math  Operator=square  SaturateOnIntegerOverflow=on
  Square2 : Math  Operator=square  SaturateOnIntegerOverflow=on
  Transpose : Math  Operator=transpose  SaturateOnIntegerOverflow=on
  Transpose1 : Math  Operator=transpose  SaturateOnIntegerOverflow=on
  "İtki Kuvveti " : Outport
  İtki Eylemsizlik Momenti : Outport  Port=2
  wires:
  Hava Yoğunluğu/1 -> Gain/1
  Gain1/1 -> Square/1
  Hava Hızı/1 -> Square1/1
  Square1/1 -> Minus/2
  Square/1 -> Minus/1
  Minus/1 -> Product/2
  Gain/1 -> Product/1
  Product/1 -> Matrix Concatenate/1
  Constant1/1 -> Matrix Concatenate/3, Matrix Concatenate/2
  Matrix Concatenate/1 -> Transpose/1
  Transpose/1 -> "İtki Kuvveti "/1
  Gain2/1 -> Square2/1
  "Pulse Input "/1 -> Gain1/1, Gain2/1
  Square2/1 -> Gain3/1
  Matrix Concatenate1/1 -> Transpose1/1
  Constant2/1 -> Matrix Concatenate1/2, Matrix Concatenate1/3
  Gain3/1 -> Matrix Concatenate1/1
  Transpose1/1 -> İtki Eylemsizlik Momenti/1

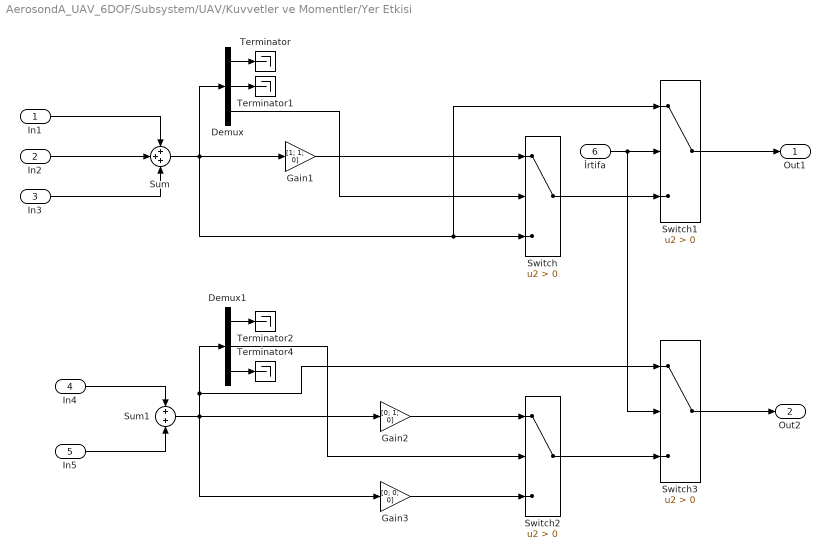
== system AerosondA_UAV_6DOF/Subsystem/UAV/Kuvvetler ve Momentler/Yer Etkisi  ==
  In1 : Inport
  In2 : Inport  Port=2
  In3 : Inport  Port=3
  In4 : Inport  Port=4
  In5 : Inport  Port=5
  "İrtifa " : Inport  Port=6
  Demux : Demux  Outputs=3
  Demux1 : Demux  Outputs=3
  Gain1 : Gain  Gain=[1; 1; 0]
  Gain2 : Gain  Gain=[0; 1; 0]
  Gain3 : Gain  Gain=[0; 0; 0]
  Sum : Sum  Inputs=+++
  Sum1 : Sum
  Switch{,1..3} (4 alike) : Switch  Criteria=u2 > Threshold
  Terminator{,1..2,4} (4 alike) : Terminator
  Out1 : Outport
  Out2 : Outport  Port=2
  wires:
  In2/1 -> Sum/2
  In1/1 -> Sum/1
  In3/1 -> Sum/3
  In4/1 -> Sum1/1
  In5/1 -> Sum1/2
  Sum/1 -> Switch1/1, Switch/3, Demux/1, Gain1/1
  Demux/1 -> Terminator/1
  Demux/2 -> Terminator1/1
  Demux/3 -> Switch/2
  Gain1/1 -> Switch/1
  Switch/1 -> Switch1/3
  Switch1/1 -> Out1/1
  Switch3/1 -> Out2/1
  Demux1/2 -> Switch2/2
  Switch2/1 -> Switch3/3
  Demux1/1 -> Terminator2/1
  "İrtifa "/1 -> Switch3/2, Switch1/2
  Demux1/3 -> Terminator4/1
  Gain3/1 -> Switch2/3
  Sum1/1 -> Gain2/1, Gain3/1, Switch3/1, Demux1/1
  Gain2/1 -> Switch2/1

== system AerosondA_UAV_6DOF/Subsystem/UAV/Kuvvetler ve Momentler/Yerçekimi Kuvveti ==
  Kütle (kg) : Inport
  Euler Matrix : Inport  Port=2
  Gain : Gain  Gain=[0; 0; 9.81]
  Matrix Multiply : Product  Multiplication=Matrix(*)
  "Yerçekimi Kuvveti " : Outport
  wires:
  Kütle (kg)/1 -> Gain/1
  Gain/1 -> Matrix Multiply/2
  Euler Matrix/1 -> Matrix Multiply/1
  Matrix Multiply/1 -> "Yerçekimi Kuvveti "/1

== system AerosondA_UAV_6DOF/Subsystem/UAV/Dinamik ve Kinematik/6 DOF Model/Gövde Eksen Takımı  ==
  "Roll Açısı " : Inport
  "Pitch Açısı " : Inport  Port=2
  "Yaw Açısı " : Inport  Port=3
  Product : Product  Inputs=3  Multiplication=Matrix(*)
  Subsystem : Subsystem
  Subsystem1 : Subsystem
  Subsystem2 : Subsystem
  "Euler Matrix " : Outport
  wires:
  "Roll Açısı "/1 -> Subsystem/1("Roll Açısı ")
  "Pitch Açısı "/1 -> Subsystem1/1("Pitch Açısı ")
  "Yaw Açısı "/1 -> Subsystem2/1("Yaw Angle ")
  Subsystem/1(Roll Matris) -> Product/1
  Subsystem1/1("Pitch Matris ") -> Product/2
  Subsystem2/1("Yaw Matris ") -> Product/3
  Product/1 -> "Euler Matrix "/1

== system AerosondA_UAV_6DOF/Subsystem/UAV/Kuvvetler ve Momentler/Aerodinamik Model/Body <-> Wind  ==
  "Kayış Açısı " : Inport
  "Hücum Açısı " : Inport  Port=2
  Hücum Açısı Değişimi : Subsystem
  Kayış Açısı : Subsystem
  Product : Product  Multiplication=Matrix(*)
  Product1 : Product  Multiplication=Matrix(*)
  "Body to Wind " : Outport
  Stability to Body : Outport  Port=2
  Wind to Body : Outport  Port=3
  wires:
  Product/1 -> "Body to Wind "/1
  Hücum Açısı Değişimi/1("Hücum Açısı Matrisi ") -> Product/2, Product1/1
  Kayış Açısı/1("Kayış Açısı Matrisi ") -> Product/1, Product1/2
  "Hücum Açısı "/1 -> Hücum Açısı Değişimi/1("Hücum Açısı ")
  "Kayış Açısı "/1 -> Kayış Açısı/1("Kayış Açısı ")
  Product1/1 -> Wind to Body/1
  Hücum Açısı Değişimi/2(Stability to Body) -> Stability to Body/1

== system AerosondA_UAV_6DOF/Subsystem/UAV/Kuvvetler ve Momentler/Aerodinamik Model/Subsystem ==
  Air Speed (V_a) : Inport
  Constant : Constant  Value=0
  Matrix Concatenate : Concatenate  NumInputs=3  Mode=Multidimensional array  ConcatenateDimension=2
  Transpose : Math  Operator=transpose  SaturateOnIntegerOverflow=on
  In Wind Frame : Outport
  wires:
  Air Speed (V_a)/1 -> Matrix Concatenate/1
  Constant/1 -> Matrix Concatenate/3, Matrix Concatenate/2
  Matrix Concatenate/1 -> Transpose/1
  Transpose/1 -> In Wind Frame/1

== system AerosondA_UAV_6DOF/Subsystem/UAV/Kuvvetler ve Momentler/Atmosfer Modeli/Subsystem ==
  "İrtifa " : Inport
  Constant : Constant  Value=216.65
  Gain : Gain  Gain=6.5/1000
  Sum : Sum  Inputs=-+
  Switch : Switch  Threshold=11000
  T_0 (K) : Constant  Value=288.15
  Sıcaklık (K) : Outport
  wires:
  "İrtifa "/1 -> Gain/1, Switch/2
  Constant/1 -> Switch/1
  T_0 (K)/1 -> Sum/2
  Gain/1 -> Sum/1
  Sum/1 -> Switch/3
  Switch/1 -> Sıcaklık (K)/1

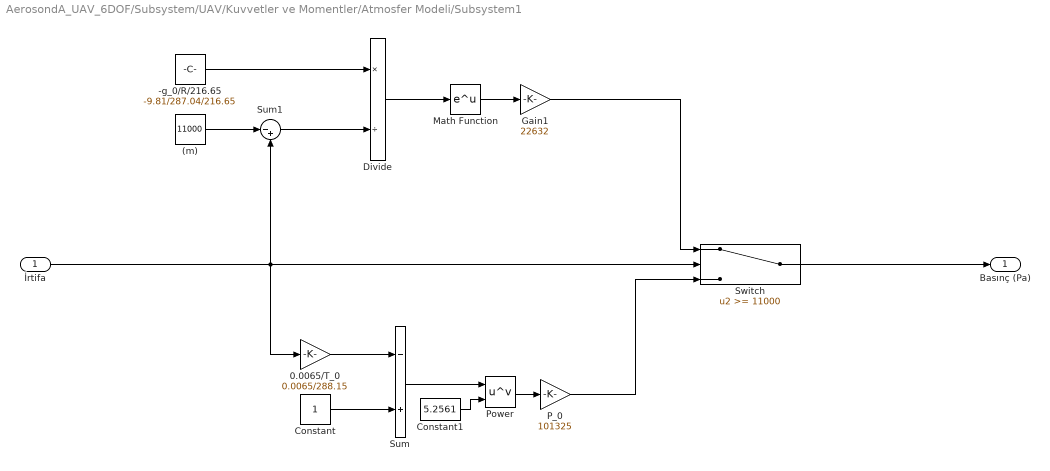
== system AerosondA_UAV_6DOF/Subsystem/UAV/Kuvvetler ve Momentler/Atmosfer Modeli/Subsystem1 ==
  "İrtifa " : Inport
  (m) : Constant  Value=11000
  -g_0/R/216.65 : Constant  Value=-9.81/287.04/216.65
  "0.0065/T_0 " : Gain  Gain=0.0065/288.15
  Constant : Constant
  Constant1 : Constant  Value=5.2561
  Divide : Product  Inputs=*/
  Gain1 : Gain  Gain=22632
  Math Function : Math  SaturateOnIntegerOverflow=on
  P_0 : Gain  Gain=101325
  Power : Math  Operator=pow  SaturateOnIntegerOverflow=on
  Sum : Sum  Inputs=-+
  Sum1 : Sum  Inputs=|-+
  Switch : Switch  Threshold=11000
  Basınç (Pa) : Outport
  wires:
  Switch/1 -> Basınç (Pa)/1
  "İrtifa "/1 -> Switch/2, "0.0065/T_0 "/1, Sum1/2
  -g_0/R/216.65/1 -> Divide/1
  Sum1/1 -> Divide/2
  (m)/1 -> Sum1/1
  Divide/1 -> Math Function/1
  Math Function/1 -> Gain1/1
  Gain1/1 -> Switch/1
  "0.0065/T_0 "/1 -> Sum/1
  Constant/1 -> Sum/2
  Sum/1 -> Power/1
  Constant1/1 -> Power/2
  Power/1 -> P_0/1
  P_0/1 -> Switch/3

== system AerosondA_UAV_6DOF/Subsystem/UAV/Kuvvetler ve Momentler/Atmosfer Modeli/Subsystem2 ==
  "Sıcaklık " : Inport
  Basınç : Inport  Port=2
  1/R : Gain  Gain=1/287.04
  Divide : Product  Inputs=/*
  Hava Yoğunluğu : Outport
  wires:
  Divide/1 -> 1/R/1
  "Sıcaklık "/1 -> Divide/1
  Basınç/1 -> Divide/2
  1/R/1 -> Hava Yoğunluğu/1

== system AerosondA_UAV_6DOF/Subsystem/UAV/Kuvvetler ve Momentler/Atmosfer Modeli/Subsystem3 ==
  "Sıcaklık " : Inport
  "Rk " : Gain  Gain=287.04*1.4
  Sqrt : Sqrt  SaturateOnIntegerOverflow=on
  Ses Hızı : Outport
  wires:
  Sqrt/1 -> Ses Hızı/1
  "Rk "/1 -> Sqrt/1
  "Sıcaklık "/1 -> "Rk "/1

== system AerosondA_UAV_6DOF/Subsystem/UAV/Kuvvetler ve Momentler/Elevator Rudder ve Aeleron/Aileron Modeli ==
  "Aileron Açısı (İstenen) " : Inport
  Command Saturation : Saturate  UpperLimit=21.5  LowerLimit=-21.5
  Gain2 : Gain  Gain=-100
  Integrator : Integrator  InitialCondition=TrimCondition(2)
  Rate Saturation : Saturate  UpperLimit=80  LowerLimit=-80
  Sum1 : Sum  Inputs=|++
  "Aileron Açısı " : Outport
  wires:
  "Aileron Açısı (İstenen) "/1 -> Command Saturation/1
  Sum1/1 -> Gain2/1
  Command Saturation/1 -> Sum1/1
  Gain2/1 -> Rate Saturation/1
  Integrator/1 -> "Aileron Açısı "/1, Sum1/2
  Rate Saturation/1 -> Integrator/1

== system AerosondA_UAV_6DOF/Subsystem/UAV/Kuvvetler ve Momentler/Elevator Rudder ve Aeleron/Elevator Modeli ==
  Elevator Açısı (İstenen) : Inport
  Command Saturation : Saturate  UpperLimit=25  LowerLimit=-25
  Gain2 : Gain  Gain=-100
  Integrator : Integrator  InitialCondition=TrimCondition(1)
  Rate Saturasyonu : Saturate  UpperLimit=60  LowerLimit=-60
  Sum1 : Sum  Inputs=|++
  Elevator Açısı : Outport
  wires:
  Sum1/1 -> Gain2/1
  Integrator/1 -> Elevator Açısı/1, Sum1/2
  Gain2/1 -> Rate Saturasyonu/1
  Rate Saturasyonu/1 -> Integrator/1
  Command Saturation/1 -> Sum1/1
  Elevator Açısı (İstenen)/1 -> Command Saturation/1

== system AerosondA_UAV_6DOF/Subsystem/UAV/Kuvvetler ve Momentler/Elevator Rudder ve Aeleron/Rudder Modeli ==
  note: Rudder Açısı (İstenen)
  Rudder Açısı (İstenen) : Inport
  Command Saturation : Saturate  UpperLimit=30  LowerLimit=-30
  Gain2 : Gain  Gain=-100
  Integrator : Integrator  InitialCondition=TrimCondition(3)
  Rate Saturation : Saturate  UpperLimit=120  LowerLimit=-120
  Sum1 : Sum  Inputs=|++
  Rudder Açısı : Outport
  wires:
  Rudder Açısı (İstenen)/1 -> Command Saturation/1
  Rate Saturation/1 -> Integrator/1
  Command Saturation/1 -> Sum1/1
  Gain2/1 -> Rate Saturation/1
  Integrator/1 -> Rudder Açısı/1, Sum1/2
  Sum1/1 -> Gain2/1

== system AerosondA_UAV_6DOF/Subsystem/UAV/Dinamik ve Kinematik/6 DOF Model/Gövde Eksen Takımı /Subsystem ==
  "Roll Açısı " : Inport
  Constant : Constant
  Constant1 : Constant  Value=0
  Constant2 : Constant  Value=0
  Constant3 : Constant  Value=0
  Cos : Trigonometry  Operator=cos
  Gain1 : Gain  Gain=-1
  Matrix Concatenate : Concatenate  NumInputs=3  Mode=Multidimensional array  ConcatenateDimension=2
  Mux : Mux  Inputs=3
  Mux1 : Mux  Inputs=3
  Mux2 : Mux  Inputs=3
  Sin : Trigonometry
  Roll Matris : Outport
  wires:
  Mux1/1 -> Matrix Concatenate/2
  "Roll Açısı "/1 -> Sin/1, Cos/1
  Matrix Concatenate/1 -> Roll Matris/1
  Sin/1 -> Mux2/2, Gain1/1
  Constant/1 -> Mux/1
  Cos/1 -> Mux2/3, Mux1/2
  Constant1/1 -> Mux/2, Mux/3
  Mux2/1 -> Matrix Concatenate/3
  Mux/1 -> Matrix Concatenate/1
  Gain1/1 -> Mux1/3
  Constant2/1 -> Mux1/1
  Constant3/1 -> Mux2/1

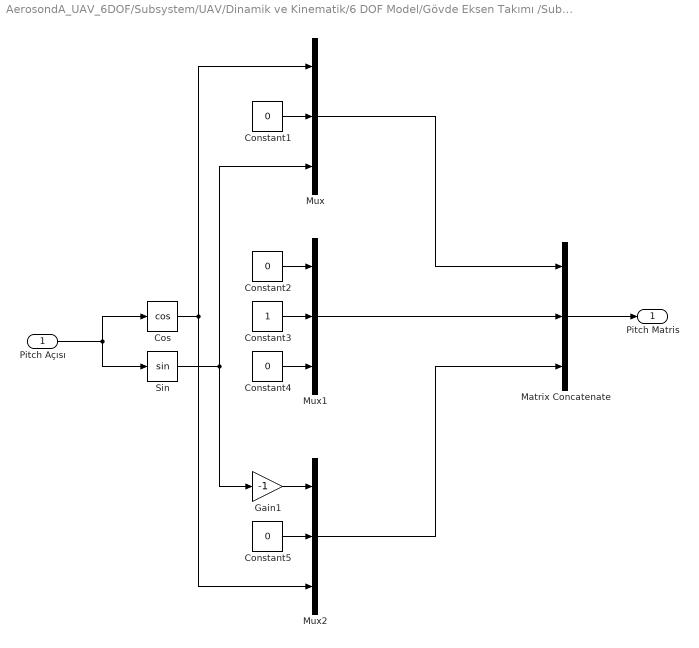
== system AerosondA_UAV_6DOF/Subsystem/UAV/Dinamik ve Kinematik/6 DOF Model/Gövde Eksen Takımı /Subsystem1 ==
  "Pitch Açısı " : Inport
  Constant{1..2,4..5} (4 alike) : Constant  Value=0
  Constant3 : Constant
  Cos : Trigonometry  Operator=cos
  Gain1 : Gain  Gain=-1
  Matrix Concatenate : Concatenate  NumInputs=3  Mode=Multidimensional array  ConcatenateDimension=2
  Mux : Mux  Inputs=3
  Mux1 : Mux  Inputs=3
  Mux2 : Mux  Inputs=3
  Sin : Trigonometry
  "Pitch Matris " : Outport
  wires:
  Mux/1 -> Matrix Concatenate/1
  Mux2/1 -> Matrix Concatenate/3
  Cos/1 -> Mux/1, Mux2/3
  Matrix Concatenate/1 -> "Pitch Matris "/1
  "Pitch Açısı "/1 -> Cos/1, Sin/1
  Mux1/1 -> Matrix Concatenate/2
  Sin/1 -> Mux/3, Gain1/1
  Constant1/1 -> Mux/2
  Constant2/1 -> Mux1/1
  Constant3/1 -> Mux1/2
  Constant4/1 -> Mux1/3
  Constant5/1 -> Mux2/2
  Gain1/1 -> Mux2/1

== system AerosondA_UAV_6DOF/Subsystem/UAV/Dinamik ve Kinematik/6 DOF Model/Gövde Eksen Takımı /Subsystem2 ==
  "Yaw Angle " : Inport
  Constant{1..4} (4 alike) : Constant  Value=0
  Constant5 : Constant
  Cos : Trigonometry  Operator=cos
  Gain2 : Gain  Gain=-1
  Matrix Concatenate : Concatenate  NumInputs=3  Mode=Multidimensional array  ConcatenateDimension=2
  Mux : Mux  Inputs=3
  Mux1 : Mux  Inputs=3
  Mux2 : Mux  Inputs=3
  Sin : Trigonometry
  "Yaw Matris " : Outport
  wires:
  Mux1/1 -> Matrix Concatenate/2
  "Yaw Angle "/1 -> Sin/1, Cos/1
  Matrix Concatenate/1 -> "Yaw Matris "/1
  Mux2/1 -> Matrix Concatenate/3
  Mux/1 -> Matrix Concatenate/1
  Cos/1 -> Mux/1, Mux1/2
  Constant1/1 -> Mux/3
  Sin/1 -> Mux1/1, Gain2/1
  Constant2/1 -> Mux1/3
  Constant3/1 -> Mux2/1
  Constant4/1 -> Mux2/2
  Constant5/1 -> Mux2/3
  Gain2/1 -> Mux/2

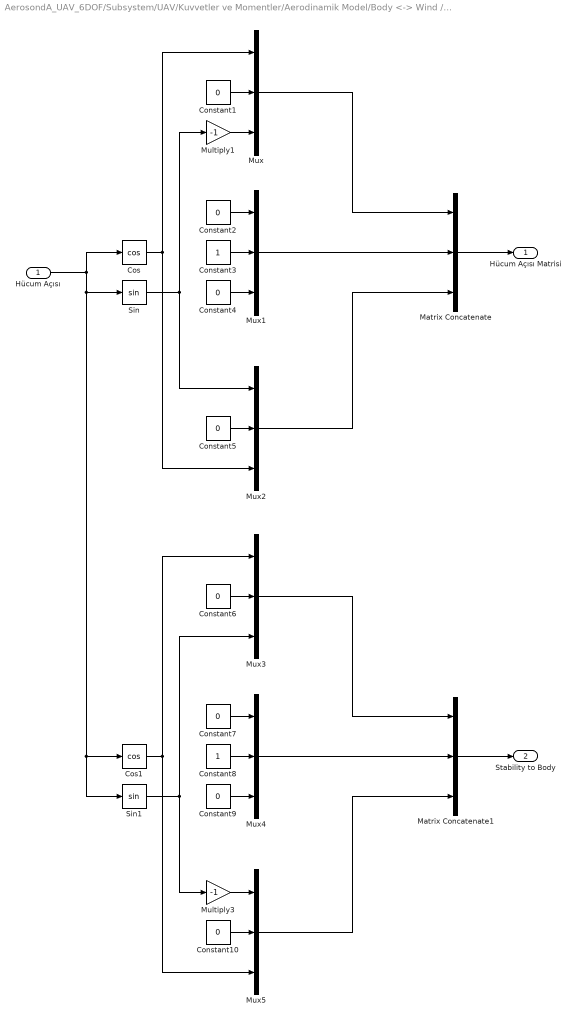
== system AerosondA_UAV_6DOF/Subsystem/UAV/Kuvvetler ve Momentler/Aerodinamik Model/Body <-> Wind /Hücum Açısı Değişimi ==
  "Hücum Açısı " : Inport
  Constant{1..2,4..7,9..10} (8 alike) : Constant  Value=0  VectorParams1D=off
  Constant3 : Constant  VectorParams1D=off
  Constant8 : Constant  VectorParams1D=off
  Cos : Trigonometry  Operator=cos
  Cos1 : Trigonometry  Operator=cos
  Matrix Concatenate : Concatenate  NumInputs=3  Mode=Multidimensional array  ConcatenateDimension=2
  Matrix Concatenate1 : Concatenate  NumInputs=3  Mode=Multidimensional array  ConcatenateDimension=2
  Multiply1 : Gain  Gain=-1
  Multiply3 : Gain  Gain=-1
  Mux{,1..5} (6 alike) : Mux  Inputs=3
  Sin : Trigonometry
  Sin1 : Trigonometry
  "Hücum Açısı Matrisi " : Outport
  Stability to Body : Outport  Port=2
  wires:
  Constant5/1 -> Mux2/2
  Constant4/1 -> Mux1/3
  Constant3/1 -> Mux1/2
  Constant2/1 -> Mux1/1
  Constant1/1 -> Mux/2
  Mux1/1 -> Matrix Concatenate/2
  Matrix Concatenate/1 -> "Hücum Açısı Matrisi "/1
  Cos/1 -> Mux2/3, Mux/1
  Mux2/1 -> Matrix Concatenate/3
  Mux/1 -> Matrix Concatenate/1
  Sin/1 -> Mux2/1, Multiply1/1
  Multiply1/1 -> Mux/3
  Sin1/1 -> Mux3/3, Multiply3/1
  Mux3/1 -> Matrix Concatenate1/1
  Mux5/1 -> Matrix Concatenate1/3
  Cos1/1 -> Mux3/1, Mux5/3
  Matrix Concatenate1/1 -> Stability to Body/1
  "Hücum Açısı "/1 -> Sin1/1, Cos1/1, Sin/1, Cos/1
  Mux4/1 -> Matrix Concatenate1/2
  Constant6/1 -> Mux3/2
  Constant7/1 -> Mux4/1
  Constant8/1 -> Mux4/2
  Constant9/1 -> Mux4/3
  Constant10/1 -> Mux5/2
  Multiply3/1 -> Mux5/1

== system AerosondA_UAV_6DOF/Subsystem/UAV/Kuvvetler ve Momentler/Aerodinamik Model/Body <-> Wind /Kayış Açısı ==
  "Kayış Açısı " : Inport
  Constant : Constant
  Constant{1..4} (4 alike) : Constant  Value=0
  Cos : Trigonometry  Operator=cos
  Gain1 : Gain  Gain=-1
  Matrix Concatenate : Concatenate  NumInputs=3  Mode=Multidimensional array  ConcatenateDimension=2
  Mux : Mux  Inputs=3
  Mux1 : Mux  Inputs=3
  Mux2 : Mux  Inputs=3
  Sin : Trigonometry
  "Kayış Açısı Matrisi " : Outport
  wires:
  Mux/1 -> Matrix Concatenate/1
  Mux2/1 -> Matrix Concatenate/3
  Matrix Concatenate/1 -> "Kayış Açısı Matrisi "/1
  "Kayış Açısı "/1 -> Cos/1, Sin/1
  Mux1/1 -> Matrix Concatenate/2
  Cos/1 -> Mux1/2, Mux/1
  Constant1/1 -> Mux/3
  Sin/1 -> Mux1/1, Gain1/1
  Constant2/1 -> Mux1/3
  Constant3/1 -> Mux2/1
  Constant4/1 -> Mux2/2
  Constant/1 -> Mux2/3
  Gain1/1 -> Mux/2
